simulink model "dp_UKF"  (R2015b)
settings: Solver=FixedStepAuto  StartTime=0.0  StopTime=5  FixedStep=T_s  RelTol=1e-3
InitFcn:
  | dp_UKF_script
values from neighbouring files (symbols this model uses):
  alpha = 0.001    [dp_UKF_script.m]
  beta = 2    [dp_UKF_script.m]
  d_p1 = 0.001    [dp_EKF_script.m]    (also in dp_UKF_script.m; dp_kalman_script.m; dp_real_vs_lin_script.m; dp_statefeedback_script.m)
  d_p2 = 0.001    [dp_EKF_script.m]    (also in dp_UKF_script.m; dp_kalman_script.m; dp_real_vs_lin_script.m; dp_statefeedback_script.m)
  g = 9.81    [dp_EKF_script.m]    (also in dp_UKF_script.m; dp_kalman_script.m; dp_real_vs_lin_script.m; dp_statefeedback_script.m)
  kappa = 0    [dp_UKF_script.m]
  l_1 = 0.194    [dp_EKF_script.m]    (also in dp_UKF_script.m; dp_kalman_script.m; dp_real_vs_lin_script.m; dp_statefeedback_script.m)
  l_2 = 0.1855    [dp_EKF_script.m]    (also in dp_UKF_script.m; dp_kalman_script.m; dp_real_vs_lin_script.m; dp_statefeedback_script.m)
  m_1 = 0.0313    [dp_EKF_script.m]    (also in dp_UKF_script.m; dp_kalman_script.m; dp_real_vs_lin_script.m; dp_statefeedback_script.m)
  m_2 = 0.0313    [dp_EKF_script.m]    (also in dp_UKF_script.m; dp_kalman_script.m; dp_real_vs_lin_script.m; dp_statefeedback_script.m)
  m_3 = 0.0308    [dp_EKF_script.m]    (also in dp_UKF_script.m; dp_kalman_script.m; dp_real_vs_lin_script.m; dp_statefeedback_script.m)
  Pk_0 = eye(4)    [dp_EKF_script.m]    (also in dp_UKF_script.m; dp_kalman_script.m = 1*eye(4); dp_real_vs_lin_script.m)
  Qk = zeros(4,4,steps,steps,steps,steps)    [dp_EKF_script.m]    (also in dp_UKF_script.m = zeros(4,4,9,9); dp_kalman_script.m = 1e-4*diag([1 1 1e-2 1e-2]); dp_real_vs_lin_script.m = 0*diag([1 1 1 1]))
  Rk = 1    [dp_EKF_script.m]    (also in dp_UKF_script.m; dp_kalman_script.m = 0.01; dp_real_vs_lin_script.m = 0.001)
  T_s = 0.001    [dp_EKF_script.m]    (also in dp_UKF_script.m; dp_kalman_script.m; dp_real_vs_lin_script.m; dp_statefeedback_script.m)
  x0 = [phi1_0; dphi1_0; phi2_0; dphi2_0]    [dp_EKF_script.m]    (also in dp_UKF_script.m; dp_kalman_script.m; dp_real_vs_lin_script.m; dp_statefeedback_script.m)
libraries: simulink x2
settings Model: Creator=serov  LastModifiedBy=serov

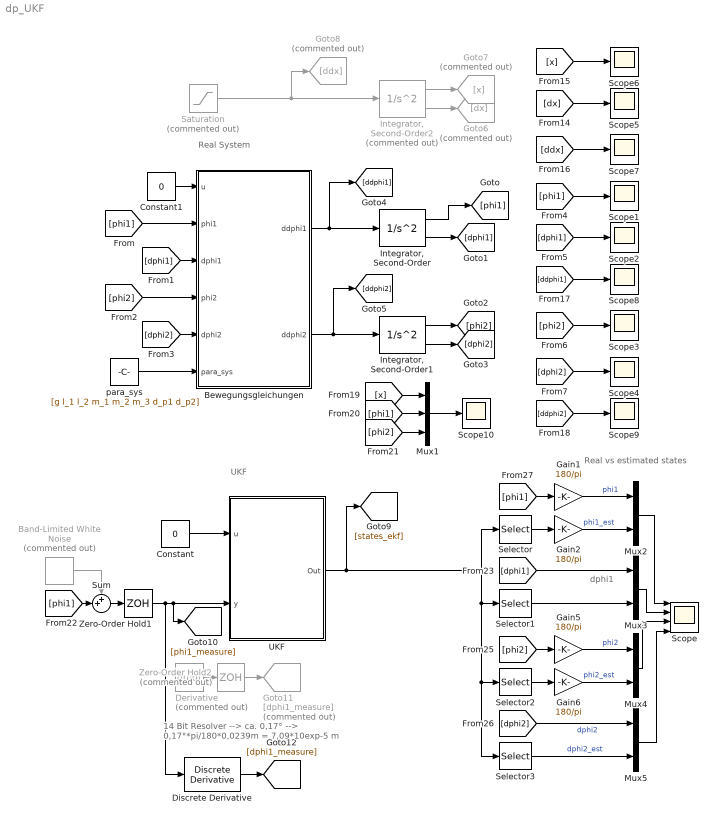
== system dp_UKF ==
  note: dphi1
  note: Real vs estimated states
  note: Real System
  note: UKF
  note: 14 Bit Resolver --> ca. 0,17°
      | --> 0,17°*pi/180*0,0239m = 7,09*10exp-5 m
  Band-Limited White Noise : simulink/Sources/Band-Limited White Noise  Commented=on  Cov=0.5*0.000000003  Ts=0.001  seed=[23341]
  Bewegungsgleichungen : MATLAB Function  TreatAsAtomicUnit=on
  Constant : Constant  Value=0  SampleTime=T_s
  Constant1 : Constant  Value=0  SampleTime=T_s
  Derivative : Derivative  Commented=on
  Discrete Derivative : simulink/Discrete/Discrete Derivative  gainval=1.0  ICPrevScaledInput=0.0  InputProcessing=Inherited  OutMin=[]  OutMax=[]  OutDataType=fixdt(1, 16)  OutScaling=2^-10  DoSatur=off
  Gain{1..2,5..6} (4 alike) : Gain  Gain=180/pi
  Goto11 : Goto  Commented=on  GotoTag=dphi1_measure
  Goto6 : Goto  Commented=on  GotoTag=dx
  Goto7 : Goto  Commented=on  GotoTag=x
  Goto8 : Goto  Commented=on  GotoTag=ddx
  "Integrator, Second-Order" : SecondOrderIntegrator  ICX=phi1_0  ICDXDT=dphi1_0
  "Integrator, Second-Order1" : SecondOrderIntegrator  ICX=phi2_0  ICDXDT=dphi2_0
  "Integrator, Second-Order2" : SecondOrderIntegrator  Commented=on  ICX=x_0  LimitX=on  UpperLimitX=0.2  LowerLimitX=-0.2  ICDXDT=dx_0  LimitDXDT=on  UpperLimitDXDT=5  LowerLimitDXDT=-5
  Mux1 : Mux  Inputs=3
  Mux{2..5} (4 alike) : Mux  Inputs=2
  Saturation : Saturate  Commented=on  UpperLimit=20  LowerLimit=-20
  Scope : Scope  NumInputPorts=4
  Scope{1..10} (10 alike) : Scope
  Selector : Selector  InputPortWidth=4  IndexOptions=Index vector (dialog)  Indices=[1]  OutputSizes=1
  Selector1 : Selector  InputPortWidth=4  IndexOptions=Index vector (dialog)  Indices=[2]  OutputSizes=1
  Selector2 : Selector  InputPortWidth=4  IndexOptions=Index vector (dialog)  Indices=[3]  OutputSizes=1
  Selector3 : Selector  InputPortWidth=4  IndexOptions=Index vector (dialog)  Indices=[4]  OutputSizes=1
  Sum : Sum  Inputs=++|
  UKF : Subsystem
  Zero-Order Hold1 : ZeroOrderHold  SampleTime=T_s
  Zero-Order Hold2 : ZeroOrderHold  Commented=on  SampleTime=T_s
  para_sys : Constant  Value=[g l_1 l_2 m_1 m_2 m_3 d_p1 d_p2]
  wires:
  Bewegungsgleichungen/1(ddphi1) -> [ddphi1], "Integrator, Second-Order"/1
  Bewegungsgleichungen/2(ddphi2) -> [ddphi2], "Integrator, Second-Order1"/1
  "Integrator, Second-Order"/2 -> [dphi1]
  "Integrator, Second-Order1"/2 -> [dphi2]
  "Integrator, Second-Order1"/1 -> [phi2]
  [phi1] -> Bewegungsgleichungen/2(phi1)
  [dphi1] -> Bewegungsgleichungen/3(dphi1)
  [phi2] -> Bewegungsgleichungen/4(phi2)
  [dphi2] -> Bewegungsgleichungen/5(dphi2)
  para_sys/1 -> Bewegungsgleichungen/6(para_sys)
  [phi1] -> Scope1/1
  [dphi1] -> Scope2/1
  [phi2] -> Scope3/1
  [dphi2] -> Scope4/1
  "Integrator, Second-Order2"/1 -> Goto7/1
  "Integrator, Second-Order2"/2 -> Goto6/1
  [dx] -> Scope5/1
  [x] -> Scope6/1
  [ddx] -> Scope7/1
  [ddphi1] -> Scope8/1
  [ddphi2] -> Scope9/1
  Saturation/1 -> Goto8/1, "Integrator, Second-Order2"/1
  Mux1/1 -> Scope10/1
  [x] -> Mux1/1
  [phi1] -> Mux1/2
  [phi2] -> Mux1/3
  Zero-Order Hold1/1 -> Discrete Derivative/1, UKF/2(y), [phi1_measure]
  [phi1] -> Gain1/1
  Gain1/1 -> Mux2/1  "phi1"
  Gain2/1 -> Mux2/2  "phi1_est"
  Selector/1 -> Gain2/1
  [dphi1] -> Mux3/1
  Selector1/1 -> Mux3/2
  [phi2] -> Gain5/1
  Gain5/1 -> Mux4/1  "phi2"
  Gain6/1 -> Mux4/2  "phi2_est"
  Selector2/1 -> Gain6/1
  [dphi2] -> Mux5/1  "dphi2"
  Selector3/1 -> Mux5/2  "dphi2_est"
  UKF/1(Out) -> Selector/1, Selector3/1, Selector2/1, Selector1/1, [states_ekf]
  Mux2/1 -> Scope/1
  Mux3/1 -> Scope/2
  Mux4/1 -> Scope/3
  Mux5/1 -> Scope/4
  [phi1] -> Sum/2
  Band-Limited White Noise/1 -> Sum/1
  Sum/1 -> Zero-Order Hold1/1
  Derivative/1 -> Zero-Order Hold2/1
  Zero-Order Hold2/1 -> Goto11/1
  "Integrator, Second-Order"/1 -> [phi1]
  Discrete Derivative/1 -> [dphi1_measure]
  Constant/1 -> UKF/1(u)
  Constant1/1 -> Bewegungsgleichungen/1(u)

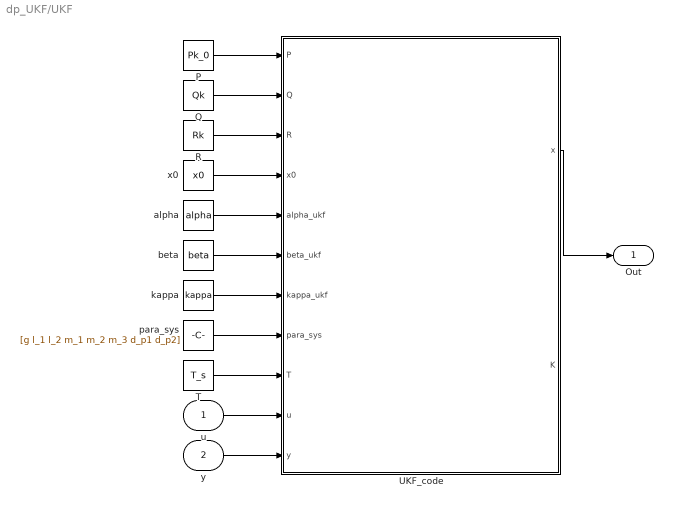
== system dp_UKF/UKF ==
  u : Inport
  y : Inport  Port=2
  P : Constant  Value=Pk_0
  Q : Constant  Value=Qk
  R : Constant  Value=Rk
  T : Constant  Value=T_s
  UKF_code : MATLAB Function  TreatAsAtomicUnit=on
  alpha : Constant  Value=alpha
  beta : Constant  Value=beta
  kappa : Constant  Value=kappa
  para_sys : Constant  Value=[g l_1 l_2 m_1 m_2 m_3 d_p1 d_p2]
  x0 : Constant  Value=x0
  Out : Outport
  wires:
  P/1 -> UKF_code/1(P)
  Q/1 -> UKF_code/2(Q)
  R/1 -> UKF_code/3(R)
  x0/1 -> UKF_code/4(x0)
  alpha/1 -> UKF_code/5(alpha_ukf)
  beta/1 -> UKF_code/6(beta_ukf)
  kappa/1 -> UKF_code/7(kappa_ukf)
  para_sys/1 -> UKF_code/8(para_sys)
  T/1 -> UKF_code/9(T)
  u/1 -> UKF_code/10(u)
  y/1 -> UKF_code/11(y)
  UKF_code/1(x) -> Out/1

== matlab function dp_UKF/UKF/UKF_code ==
  data: P input; Q input; R input; x0 input; alpha_ukf input; beta_ukf input; kappa_ukf input; para_sys input; T input; u input; y input; x output; K output
function [x,K] = unscented_kalman_filter(P, Q, R, x0, alpha_ukf, beta_ukf, kappa_ukf, para_sys, T, u, y)
% Unscented Kalman Filter (UKF) fuer nichtlineare Systeme
% Das UKF praediziert den Zustand eines nichtliniearen Systems durch
% Mittelung sog. Sigma Punkte. Dazu werden 2n+1 Sigmapunkte (moegliche
% Zustaende des Systems) mittels Kovarianzmatrix P berechnet und fuer jeden
% Sigmapunkt mithilfe der Zustandsgleichung ein neuer Zustand praediziert.
% Diese werden gewichtet gemittelt und mit deren Hilfe die neuen
% Kovarianzmatrizen, die Rueckfuehrmatrix K und die Zustaende ermittelt.
% Weitere Infos unter
% http://www.agnld.uni-potsdam.de/~shw/TSA/Tools/UKF/node4.html
% http://cslu.cse.ogi.edu/nsel/ukf/node6.html
%
% Tipp: kappa meist zu 0 waehlen, alpha sehr klein bspw. 0.001, beta bei
% Gaussverteilung = 2
% -alpha bestimmt die Streuung der Sigma-Punkte um den Mittelwert
% -beta wird benutzt, um Wissen ueber die Verteilung aufzunehmen
% -kappa ist ein sekundaerer skalierender Parameter, der gewoehnlich 
% gleich 0 oder 3-n gesetzt wird
%
% Vorlage von Matthias Dagen, September 2009, veraendert durch David
% Klinkenbuss

persistent x_p P_p x0_sig x_sig W_m W_c

% Parameter

g = para_sys(1);
l_1 = para_sys(2);
l_2 = para_sys(3);
m_1 = para_sys(4);
m_2 = para_sys(5);
m_3 = para_sys(6);
d_p1 = para_sys(7);
d_p2 = para_sys(8);

n_ukf  = 4;     % Laenge von f(x)
o_ukf = 1;      % Anzahl der zurueckgefuehrten Variablen

if isempty(x_p) || isempty(P_p) || isempty(x0_sig) || isempty(x_sig) || isempty(W_m) || isempty(W_c)
    x_p = x0;
    P_p = P;
    x0_sig = zeros(n_ukf,2*n_ukf+1);
    x_sig  = zeros(n_ukf,2*n_ukf+1);
    W_m = zeros(1,2*n_ukf+1);
    W_c = zeros(1,2*n_ukf+1);
    x = x_p;
    K = zeros(4,1);
else

%% Parameter-Initialization
lambda_ukf = (alpha_ukf^2)*(n_ukf+kappa_ukf)-n_ukf;

%% Weight calculation
W_m(1,1) = lambda_ukf/(n_ukf+lambda_ukf);
W_c(1,1) = lambda_ukf/(n_ukf+lambda_ukf)+1-alpha_ukf^2+beta_ukf;
for i=2:2*n_ukf+1
    W_m(1,i) = 1/(2*(n_ukf+lambda_ukf));
    W_c(1,i) = 1/(2*(n_ukf+lambda_ukf));
end

%% 2n+1 Sigma Points calculation

P_an = (sqrt(n_ukf+lambda_ukf).*chol(P_p))'; % Wurzelmatrix mittels Cholesky-Zerlegung
x0_sig(:,1) = x_p;
for i=2:n_ukf+1
    x0_sig(:,i)     = x_p + P_an(:,i-1);
    x0_sig(:,n_ukf+i)   = x_p - P_an(:,i-1);
end

%% Unscented Kalman filter time update equations
for i = 1:(2*n_ukf+1)


 x_1 = x0_sig(1,i);
 x_2 = x0_sig(2,i);
 x_3 = x0_sig(3,i);
 x_4 = x0_sig(4,i);

x_sig(:,i) = [x_1 + T*x_2;x_2 + (T*(12*d_p2*l_2*x_4 - 12*d_p1*l_2*x_2 - 12*d_p2*l_2*x_2 - cos(x_1 - x_3)*(18*d_p2*l_1*x_2 - 18*d_p2*l_1*x_4 + 9*l_1*l_2*m_2*u*cos(x_3) + 9*g*l_1*l_2*m_2*sin(x_3) + 9*l_1^2*l_2*m_2*x_2^2*sin(x_1 - x_3)) + 6*l_1*l_2*m_1*u*cos(x_1) + 12*l_1*l_2*m_2*u*cos(x_1) + 12*l_1*l_2*m_3*u*cos(x_1) + 6*g*l_1*l_2*m_1*sin(x_1) + 12*g*l_1*l_2*m_2*sin(x_1) + 12*g*l_1*l_2*m_3*sin(x_1) - 6*l_1*l_2^2*m_2*x_4^2*sin(x_1 - x_3)))/(l_1^2*l_2*(4*m_1 + 12*m_2 + 12*m_3 - 9*m_2*cos(x_1 - x_3)^2));x_3 + T*x_4;x_4 + (T*(sin(x_1 - x_3)*(36*l_1^2*l_2*m_2^2*x_2^2 + 12*l_1^2*l_2*m_1*m_2*x_2^2 + 36*l_1^2*l_2*m_2*m_3*x_2^2) + 24*d_p2*l_1*m_1*x_2 + 72*d_p2*l_1*m_2*x_2 - 24*d_p2*l_1*m_1*x_4 + 72*d_p2*l_1*m_3*x_2 - 72*d_p2*l_1*m_2*x_4 - 72*d_p2*l_1*m_3*x_4 + 36*d_p1*l_2*m_2*x_2*cos(x_1 - x_3) + 36*d_p2*l_2*m_2*x_2*cos(x_1 - x_3) - 36*d_p2*l_2*m_2*x_4*cos(x_1 - x_3) + 18*l_1*l_2*m_2^2*u*cos(x_3) + 18*g*l_1*l_2*m_2^2*sin(x_3) + 9*l_1*l_2^2*m_2^2*x_4^2*sin(2*x_1 - 2*x_3) - 18*l_1*l_2*m_2^2*u*cos(2*x_1 - x_3) - 18*g*l_1*l_2*m_2^2*sin(2*x_1 - x_3) + 3*l_1*l_2*m_1*m_2*u*cos(x_3) + 18*l_1*l_2*m_2*m_3*u*cos(x_3) + 3*g*l_1*l_2*m_1*m_2*sin(x_3) + 18*g*l_1*l_2*m_2*m_3*sin(x_3) - 9*l_1*l_2*m_1*m_2*u*cos(2*x_1 - x_3) - 18*l_1*l_2*m_2*m_3*u*cos(2*x_1 - x_3) - 9*g*l_1*l_2*m_1*m_2*sin(2*x_1 - x_3) - 18*g*l_1*l_2*m_2*m_3*sin(2*x_1 - x_3)))/(l_1*l_2^2*m_2*(8*m_1 + 15*m_2 + 24*m_3 - 9*m_2*cos(2*x_1 - 2*x_3)))];

end
y_sig= [1 0 0 0] * x_sig;
% Prediction, weighted sum
x_p  = x_sig * W_m';
y_  = y_sig * W_m';
%P_p calculation
P_p = P_p .* 0;
for i=1:(2*n_ukf+1)
    P_p = P_p + ((x_sig(:,i) - x_p) * (x_sig(:,i) - x_p)' .* W_c(1,i));
end
P_p  = P_p + Q;

%% Unscented Kalman filter measurement update equations
% Pyy calculation
P_yy = zeros(o_ukf,o_ukf);
for i=1:(2*n_ukf+1)
    P_yy = P_yy + ((y_sig(:,i) - y_) * (y_sig(:,i) - y_)' .* W_c(1,i));
end
P_yy = P_yy + R;
% Pxy calculation
P_xy = zeros(n_ukf,o_ukf);
for i=1:(2*n_ukf+1)
    P_xy = P_xy+((x_sig(:,i)-x_p)*(y_sig(:,i)-y_)'.*W_c(1,i));
end
% Kalman Gain
K  = P_xy/(P_yy);
P_p = P_p - (K * P_yy * K');
x  = x_p +  K * ( y - y_);
x_p = x;
end

== matlab function dp_UKF/Bewegungsgleichungen ==
  data: u input; phi1 input; dphi1 input; phi2 input; dphi2 input; para_sys input; ddphi1 output; ddphi2 output
function [ddphi1, ddphi2] = pendel_1_2(u, phi1, dphi1, phi2, dphi2, para_sys)
%#codegen

g = para_sys(1);
l_1 = para_sys(2);
l_2 = para_sys(3);
m_1 = para_sys(4);
m_2 = para_sys(5);
m_3 = para_sys(6);
d_p1 = para_sys(7);
d_p2 = para_sys(8);

ddphi1 = 1/(l_1^2*(9*cos(phi1-phi2)^2*m_2-4*m_1-12*m_2-12*m_3)*l_2)*(9*dphi1^2*cos(phi1-phi2)*sin(phi1-phi2)*l_1^2*l_2*m_2+6*m_2*l_1*l_2^2*sin(phi1-phi2)*dphi2^2+9*u*cos(phi1-phi2)*cos(phi2)*l_1*l_2*m_2+9*cos(phi1-phi2)*sin(phi2)*g*l_1*l_2*m_2-6*l_1*cos(phi1)*u*m_1*l_2-12*l_1*cos(phi1)*u*m_2*l_2-12*l_1*cos(phi1)*u*m_3*l_2-6*l_1*g*sin(phi1)*m_1*l_2-12*l_1*g*sin(phi1)*m_2*l_2-12*l_1*g*sin(phi1)*m_3*l_2+18*dphi1*cos(phi1-phi2)*d_p2*l_1-18*dphi2*cos(phi1-phi2)*d_p2*l_1+12*dphi1*d_p1*l_2+12*dphi1*d_p2*l_2-12*d_p2*dphi2*l_2);

ddphi2 = -1/(l_1*l_2^2*(9*cos(phi1-phi2)^2*m_2-4*m_1-12*m_2-12*m_3)*m_2)*(12*dphi1*d_p2*l_1*m_1+36*dphi1*d_p2*l_1*m_2+36*dphi1*d_p2*l_1*m_3-12*dphi2*d_p2*l_1*m_1-36*dphi2*d_p2*l_1*m_2-36*dphi2*d_p2*l_1*m_3-9*cos(phi1)*u*cos(phi1-phi2)*l_1*l_2*m_1*m_2-18*cos(phi1)*u*cos(phi1-phi2)*l_1*l_2*m_2*m_3-9*cos(phi1-phi2)*sin(phi1)*g*l_1*l_2*m_1*m_2-18*cos(phi1-phi2)*sin(phi1)*g*l_1*l_2*m_2*m_3+9*dphi2^2*cos(phi1-phi2)*sin(phi1-phi2)*l_1*l_2^2*m_2^2+ 6*dphi1^2*sin(phi1-phi2)*l_1^2*l_2*m_1*m_2+ 18*dphi1^2*sin(phi1-phi2)*l_1^2*l_2*m_2*m_3-18*cos(phi1)*u*cos(phi1-phi2)*l_1*l_2*m_2^2-18*cos(phi1-phi2)*sin(phi1)*g*l_1*l_2*m_2^2 +6*u*cos(phi2)*l_1*l_2*m_1*m_2+18*u*cos(phi2)*l_1*l_2*m_2*m_3+6*sin(phi2)*g*l_1*l_2*m_1*m_2+18*sin(phi2)*g*l_1*l_2*m_2*m_3 + 18*(dphi1)^2*sin(phi1-phi2)*l_1^2*l_2*m_2^2+18*u*cos(phi2)*l_1*l_2*m_2^2+18*sin(phi2)*g*l_1*l_2*m_2^2+18*dphi1*cos(phi1-phi2)*d_p1*l_2*m_2 + 18*dphi1*cos(phi1-phi2)*d_p2*l_2*m_2-18*dphi2*cos(phi1-phi2)*d_p2*l_2*m_2);
